simulink model "HW_1_v2_2019a"  (R2019a)
settings: Solver=VariableStepAuto  StartTime=0.0  StopTime=70  RelTol=1e-12
model workspace (MAT data in the model file):
  d_tar = 20
values from neighbouring files (symbols this model uses):
  d_0 = 8    [acc1.m]
  t_H_tar = 1    [acc1.m]
  v_H0 = 28    [acc1.m]
  v_L0 = 36    [acc1.m]
  v_tar = 36    [acc1.m]
  x_H0 = 0    [acc1.m]
  x_L0 = 50    [acc1.m]
libraries: simulink x4, cstblocks x3, fl_lib x1
settings Model: Creator=jake  LastModifiedBy=chris
settings DebuggingCC: SFMachineParentedDataDiag=error

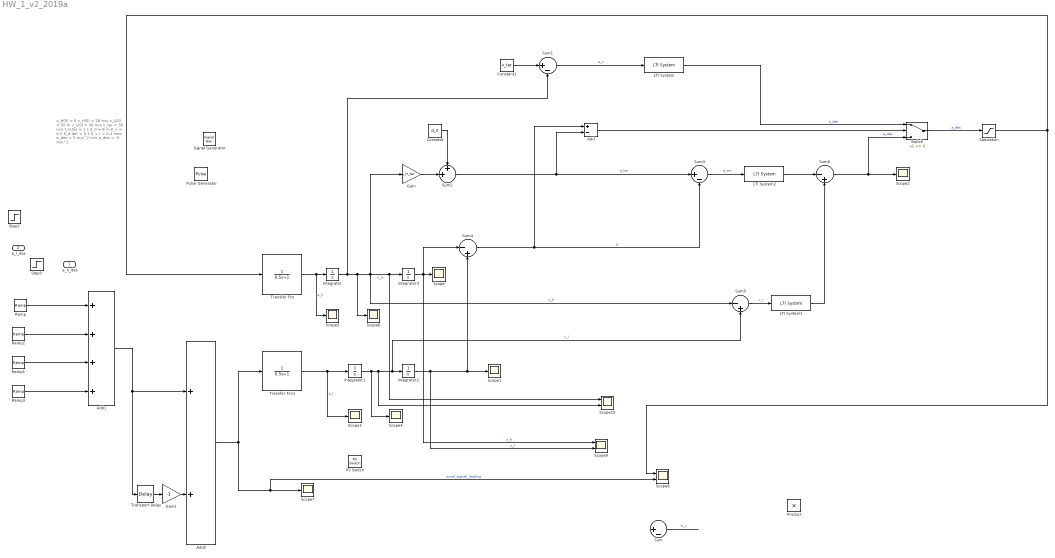
== system HW_1_v2_2019a ==
  note: x_H(0) = 0
      | v_H(0) = 28 m/s
      |
      | x_L(0) = 50 m
      | v_L(0) = 36 m/s
      |
      | v_tar = 36 m/s
      | t_H,tar = 1 s
      | d_0 = 8 m
      |
      | K_v = 0.5
      | K_d,der = 0.2
      | K_v,r = 0.4
      |
      | max a_des = 5 m/s^2
      | min a_des = -3 m/s^2
  note: v_h
  a_h_des : Inport
  a_l_des : Inport  Port=2
  Add : Sum  Inputs=+-
  Add1 : Sum  Inputs=++++
  Add2 : Sum
  Constant : Constant  Value=d_0
  Constant1 : Constant  Value=v_tar
  Gain : Gain  Gain=t_H_tar
  Gain1 : Gain  Gain=-1
  Integrator : Integrator  InitialCondition=v_H0
  Integrator1 : Integrator  InitialCondition=v_L0
  Integrator2 : Integrator  InitialCondition=x_L0
  Integrator3 : Integrator  InitialCondition=x_H0
  LTI System : cstblocks/LTI System  sys=K_v  IC=[]
  LTI System1 : cstblocks/LTI System  sys=K_v_r  IC=[]
  LTI System2 : cstblocks/LTI System  sys=K_d_err  IC=[]
  PS Switch : fl_lib/Physical Signals/Nonlinear Operators/PS Switch  Threshold=0.5
      settings: SourceProductBaseCode=SS  InternalSimscapePortConfiguration="{\"Bottom\":[],\"Left\":[{\"id\":\"I1\",\"label\":\"\",\"type\":\"input\"},{\"id\":\"I2\",\"label\":\"\",\"type\":\"input\"},{\"id\":\"I3\",\"label\":\"\",\"type\":\"input\"}],\"Right\":[{\"id\":\"O\",\"label\":\"\",\"type\":\"output\"}],\"Top\":[]}"
  Product : Product
  Pulse Generator : DiscretePulseGenerator  PulseType=Time based  Period=10  PulseWidth=5
  Ramp : simulink/Sources/Ramp  slope=-4  start=10  InitialOutput=0
  Ramp1 : simulink/Sources/Ramp  slope=4  start=13.5  InitialOutput=0
  Ramp2 : simulink/Sources/Ramp  slope=+4  start=10.5  InitialOutput=0
  Ramp3 : simulink/Sources/Ramp  slope=-4  start=14  InitialOutput=0
  Saturation : Saturate  UpperLimit=5  LowerLimit=-3
  Scope{,1..7} (8 alike) : Scope
  Scope10 : Scope  NumInputPorts=2
  Scope8 : Scope  NumInputPorts=2
  Scope9 : Scope  NumInputPorts=2
  Signal Generator : SignalGenerator  Units=rad/sec
  Step2 : Step  Time=40  After=2  SampleTime=0
  Step3 : Step  Time=43.5  After=-2  SampleTime=0
  Sum : Sum  Inputs=|+-
  Sum1 : Sum  Inputs=|+-
  Sum2 : Sum  Inputs=++|
  Sum3 : Sum  Inputs=|+-
  Sum4 : Sum  Inputs=|-+
  Sum5 : Sum  Inputs=|-+
  Sum6 : Sum  Inputs=|-+
  Switch : Switch
  Transfer Fcn : TransferFcn  Denominator=[0.5 1]
  Transfer Fcn1 : TransferFcn  Denominator=[0.5 1]
  Transport Delay : TransportDelay  DelayTime=30
  wires:
  Transfer Fcn/1 -> Scope5/1, Integrator/1  "a_h"
  Transfer Fcn1/1 -> Scope3/1, Integrator1/1  "a_l"
  Integrator1/1 -> Scope4/1, Scope10/2, Sum5/2, Integrator2/1  "v_l"
  Integrator/1 -> Sum1/2, Scope6/1, Sum5/1, Scope10/1, Integrator3/1, Gain/1  "v_h"
  Integrator2/1 -> Scope9/2, Scope1/1, Sum4/2  "x_l"
  Integrator3/1 -> Scope9/1, Sum4/1, Scope/1  "x_h"
  ? -> Sum/1  "v_tar"
  ? -> Sum/2  "v_h"
  Sum/1 -> ?  "e_v"
  Sum1/1 -> LTI System/1  "e_v"
  Gain/1 -> Sum2/2
  Constant/1 -> Sum2/1
  Sum2/1 -> Add/2, Sum3/1  "d_tar"
  Sum4/1 -> Add/1, Sum3/2  "d"
  Sum5/1 -> LTI System1/1  "v_r"
  Sum3/1 -> LTI System2/1  "d_err"
  LTI System1/1 -> Sum6/2
  LTI System2/1 -> Sum6/1
  Sum6/1 -> Switch/3, Scope2/1  "a_des"
  LTI System/1 -> Switch/1  "a_des"
  Constant1/1 -> Sum1/1
  Switch/1 -> Saturation/1  "a_des"
  Ramp/1 -> Add1/1
  Ramp2/1 -> Add1/2
  Ramp1/1 -> Add1/3
  Ramp3/1 -> Add1/4
  Add1/1 -> Transport Delay/1, Add2/1
  Add2/1 -> Scope8/2, Scope7/1, Transfer Fcn1/1  "accel_signall_leading"
  Transport Delay/1 -> Gain1/1
  Gain1/1 -> Add2/2
  Saturation/1 -> Scope8/1, Transfer Fcn/1
  Add/1 -> Switch/2
